simulink model "d"  (R2022b)
settings: Solver=ode4  StartTime=0.0  StopTime=inf  FixedStep=0.002  RelTol=1e-3
InitFcn:
  | init; % init script
values from neighbouring files (symbols this model uses):
  attitude_m0 = [theta_m0; psi_m0]    [init.m]
  attitude_t0 = [theta_t0; psi_t0]    [init.m]
  d_state_m = T_VG_m'*[V_m0;0;0;]    [init.m]
  d_state_t = T_VG_t'*[V_t0;0;0;]    [init.m]
  K_epsilon = k_LOS(1)    [init.m]
  K_sigma = k_LOS(1)    [init.m]
  state_m0 = [x_m0; y_m0; z_m0]    [init.m]
  state_t0 = [x_t0; y_t0; z_t0]    [init.m]
libraries: simulink x1
settings Model: Creator=Ali  LastModifiedBy=Ali

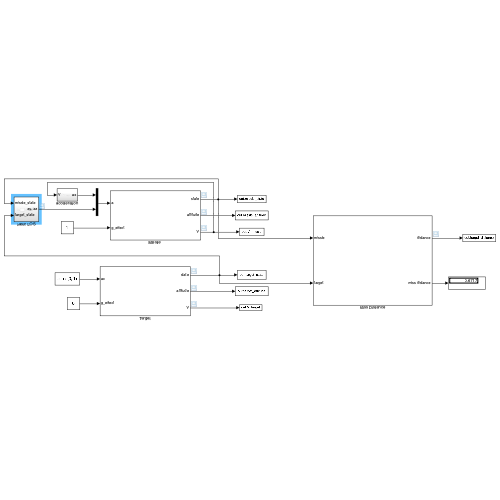
[thumbnail: Simulink's stored preview of the top-level diagram]
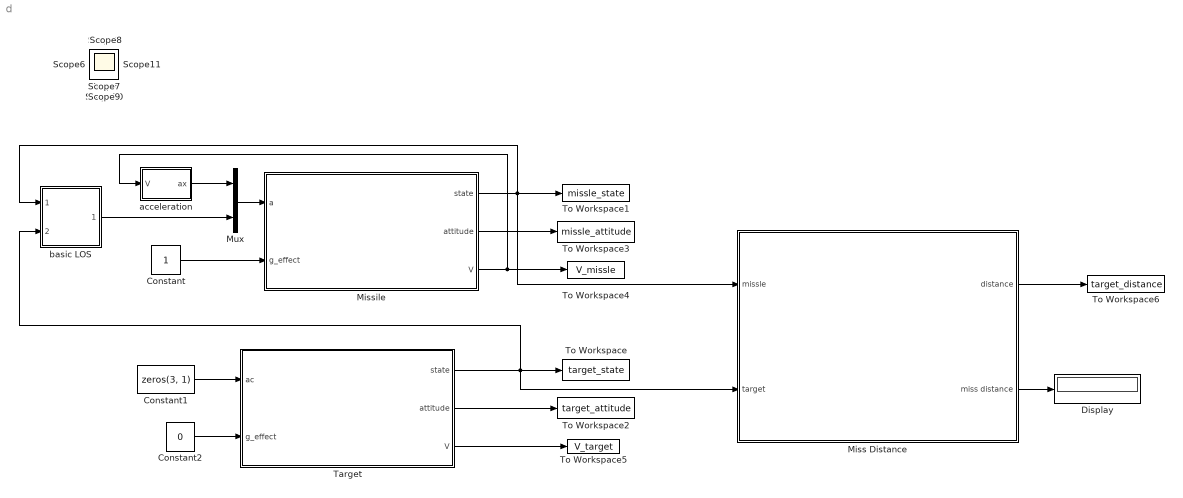
== system d ==
  Constant : Constant
  Constant1 : Constant  Value=zeros(3, 1)
  Constant2 : Constant  Value=0
  Display : Display
  Miss Distance : Subsystem
  "Missile " : Subsystem
  Mux : Mux  Inputs=2
  Target : Subsystem
  To Workspace : ToWorkspace  VariableName=target_state  SaveFormat=Timeseries  SampleTime=-1
      settings: Save2DSignal=2-D array (concatenate along first dimension)
  To Workspace1 : ToWorkspace  VariableName=missle_state  SaveFormat=Timeseries  SampleTime=-1
      settings: Save2DSignal=2-D array (concatenate along first dimension)
  To Workspace2 : ToWorkspace  VariableName=target_attitude  SaveFormat=Timeseries  SampleTime=-1
      settings: Save2DSignal=2-D array (concatenate along first dimension)
  To Workspace3 : ToWorkspace  VariableName=missle_attitude  SaveFormat=Timeseries  SampleTime=-1
      settings: Save2DSignal=2-D array (concatenate along first dimension)
  To Workspace4 : ToWorkspace  VariableName=V_missle  SaveFormat=Timeseries  SampleTime=-1
      settings: Save2DSignal=2-D array (concatenate along first dimension)
  To Workspace5 : ToWorkspace  VariableName=V_target  SaveFormat=Timeseries  SampleTime=-1
      settings: Save2DSignal=2-D array (concatenate along first dimension)
  To Workspace6 : ToWorkspace  VariableName=target_distance  SaveFormat=Timeseries  SampleTime=-1
      settings: Save2DSignal=2-D array (concatenate along first dimension)
  acceleration : Subsystem
  basic LOS : Subsystem
  Scope{,1,6..11} (8 alike) : Scope
  wires:
  Constant/1 -> "Missile "/2(g_effect)
  "Missile "/3(V) -> acceleration/1(V), To Workspace4/1
  Constant1/1 -> Target/1(ac)
  Constant2/1 -> Target/2(g_effect)
  "Missile "/1(state) -> basic LOS/1(missle_state), Miss Distance/1(missle), To Workspace1/1
  "Missile "/2(attitude) -> To Workspace3/1
  Target/1(state) -> basic LOS/2(target_state), Miss Distance/2(target), To Workspace/1
  Target/2(attitude) -> To Workspace2/1
  Target/3(V) -> To Workspace5/1
  Miss Distance/1(distance) -> To Workspace6/1
  Miss Distance/2(miss distance) -> Display/1
  acceleration/1(ax) -> Mux/1
  basic LOS/1("ay, az") -> Mux/2
  Mux/1 -> "Missile "/1(a)

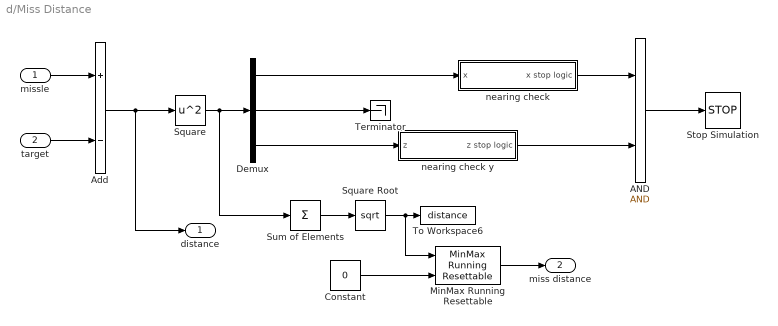
== system d/Miss Distance ==
  missle : Inport
  target : Inport  Port=2
  AND : Logic  IconShape=distinctive  AllPortsSameDT=off  OutDataTypeStr=boolean
  Add : Sum  Inputs=+-
  Constant : Constant  Value=0
  Demux : Demux  Outputs=3
  MinMax Running Resettable : simulink/Math Operations/MinMax Running Resettable  Function=min  vinit=inf
  Square : Math  Operator=square
  Square Root : Sqrt
  Stop Simulation : Stop
  Sum of Elements : Sum  Inputs=+
  Terminator : Terminator
  To Workspace6 : ToWorkspace  VariableName=distance  SaveFormat=Timeseries  SampleTime=-1
      settings: Save2DSignal=2-D array (concatenate along first dimension)
  nearing check : Subsystem
  nearing check y : Subsystem
  distance : Outport
  miss distance : Outport  Port=2
  wires:
  missle/1 -> Add/1
  Add/1 -> distance/1, Square/1
  target/1 -> Add/2
  Square/1 -> Sum of Elements/1, Demux/1
  nearing check/1(x stop logic) -> AND/1
  AND/1 -> Stop Simulation/1
  Demux/2 -> Terminator/1
  nearing check y/1(z stop logic) -> AND/2
  Sum of Elements/1 -> Square Root/1
  Square Root/1 -> MinMax Running Resettable/1, To Workspace6/1
  Demux/3 -> nearing check y/1(z)
  Demux/1 -> nearing check/1(x)
  Constant/1 -> MinMax Running Resettable/2
  MinMax Running Resettable/1 -> miss distance/1

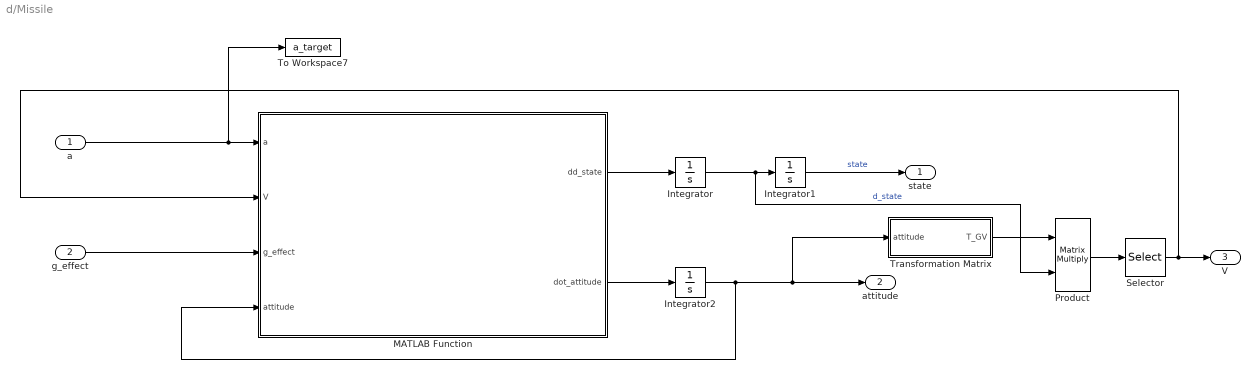
== system d/Missile  ==
  a : Inport
  g_effect : Inport  Port=2
  Integrator : Integrator  InitialCondition=d_state_m
  Integrator1 : Integrator  InitialCondition=state_m0
  Integrator2 : Integrator  InitialCondition=attitude_m0
  MATLAB Function : MATLAB Function  TreatAsAtomicUnit=on
  Product : Product  Multiplication=Matrix(*)
  Selector : Selector  InputPortWidth=3  IndexOptions=Index vector (dialog)  Indices=[1]  OutputSizes=1
  To Workspace7 : ToWorkspace  VariableName=a_target  SampleTime=-1
  Transformation Matrix : MATLAB Function  TreatAsAtomicUnit=on
  state : Outport
  attitude : Outport  Port=2
  V : Outport  Port=3
  wires:
  MATLAB Function/2(dot_attitude) -> Integrator2/1
  Integrator1/1 -> state/1  "state"
  MATLAB Function/1(dd_state) -> Integrator/1
  g_effect/1 -> MATLAB Function/3(g_effect)
  Integrator/1 -> Product/2, Integrator1/1  "d_state"
  Product/1 -> Selector/1
  Selector/1 -> MATLAB Function/2(V), V/1
  Transformation Matrix/1(T_GV) -> Product/1
  Integrator2/1 -> Transformation Matrix/1(attitude), attitude/1, MATLAB Function/4(attitude)
  a/1 -> To Workspace7/1, MATLAB Function/1(a)

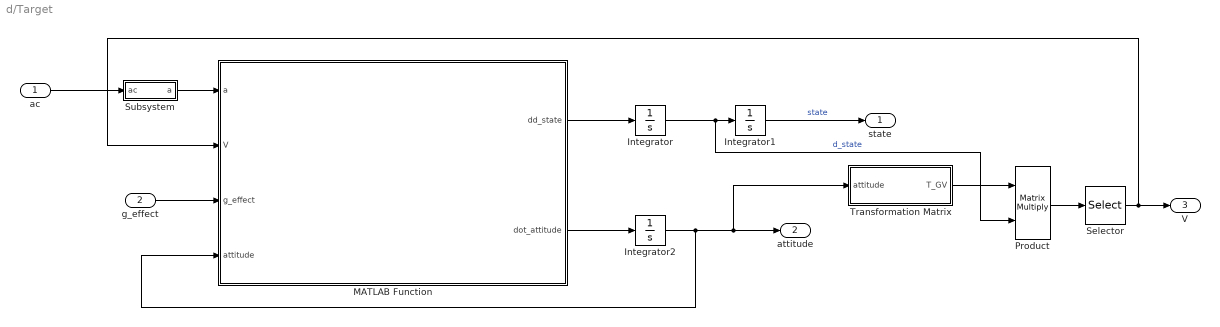
== system d/Target ==
  ac : Inport
  g_effect : Inport  Port=2
  Integrator : Integrator  InitialCondition=d_state_t
  Integrator1 : Integrator  InitialCondition=state_t0
  Integrator2 : Integrator  InitialCondition=attitude_t0
  MATLAB Function : MATLAB Function  TreatAsAtomicUnit=on
  Product : Product  Multiplication=Matrix(*)
  Selector : Selector  InputPortWidth=3  IndexOptions=Index vector (dialog)  Indices=[1]  OutputSizes=1
  Subsystem : Subsystem
  Transformation Matrix : MATLAB Function  TreatAsAtomicUnit=on
  state : Outport
  attitude : Outport  Port=2
  V : Outport  Port=3
  wires:
  MATLAB Function/2(dot_attitude) -> Integrator2/1
  Integrator1/1 -> state/1  "state"
  MATLAB Function/1(dd_state) -> Integrator/1
  g_effect/1 -> MATLAB Function/3(g_effect)
  Integrator/1 -> Product/2, Integrator1/1  "d_state"
  Integrator2/1 -> MATLAB Function/4(attitude), Transformation Matrix/1(attitude), attitude/1
  Product/1 -> Selector/1
  Selector/1 -> MATLAB Function/2(V), V/1
  Transformation Matrix/1(T_GV) -> Product/1
  ac/1 -> Subsystem/1(ac)
  Subsystem/1(a) -> MATLAB Function/1(a)

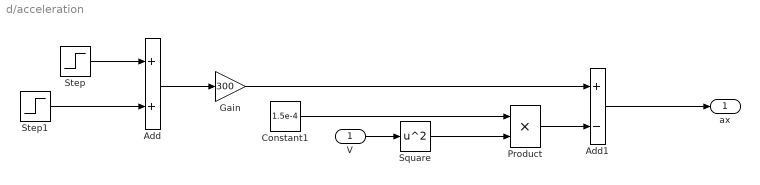
== system d/acceleration ==
  V : Inport
  Add : Sum
  Add1 : Sum  Inputs=+-
  Constant1 : Constant  Value=1.5e-4
  Gain : Gain  Gain=300
  Product : Product
  Square : Math  Operator=square
  Step : Step  Time=3  After=-1  SampleTime=0
  Step1 : Step  Time=0  SampleTime=0
  ax : Outport
  wires:
  V/1 -> Square/1
  Step/1 -> Add/1
  Square/1 -> Product/2
  Constant1/1 -> Product/1
  Add1/1 -> ax/1
  Step1/1 -> Add/2
  Gain/1 -> Add1/1
  Add/1 -> Gain/1
  Product/1 -> Add1/2

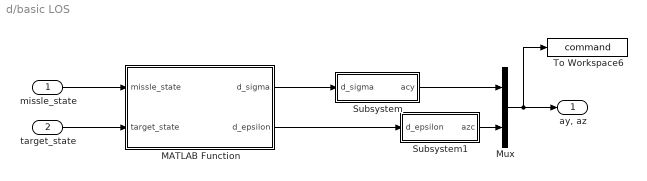
== system d/basic LOS ==
  missle_state : Inport
  target_state : Inport  Port=2
  MATLAB Function : MATLAB Function  TreatAsAtomicUnit=on
  Mux : Mux  Inputs=2
  Subsystem : Subsystem
  Subsystem1 : Subsystem
  To Workspace6 : ToWorkspace  VariableName=command  SaveFormat=Timeseries  SampleTime=-1
      settings: Save2DSignal=2-D array (concatenate along first dimension)
  "ay, az" : Outport
  wires:
  missle_state/1 -> MATLAB Function/1(missle_state)
  Mux/1 -> To Workspace6/1, "ay, az"/1
  target_state/1 -> MATLAB Function/2(target_state)
  MATLAB Function/1(d_sigma) -> Subsystem/1(d_sigma)
  Subsystem/1(acy) -> Mux/1
  MATLAB Function/2(d_epsilon) -> Subsystem1/1(d_epsilon)
  Subsystem1/1(azc) -> Mux/2

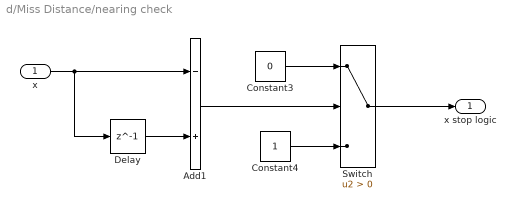
== system d/Miss Distance/nearing check ==
  x : Inport
  Add1 : Sum  Inputs=-+
  Constant3 : Constant  Value=0
  Constant4 : Constant
  Delay : Delay  DelayLength=1  InitialCondition=inf
  Switch : Switch  Criteria=u2 > Threshold  SaturateOnIntegerOverflow=off  InputSameDT=off
  x stop logic : Outport
  wires:
  Switch/1 -> x stop logic/1
  Constant3/1 -> Switch/1
  Constant4/1 -> Switch/3
  x/1 -> Delay/1, Add1/1
  Add1/1 -> Switch/2
  Delay/1 -> Add1/2

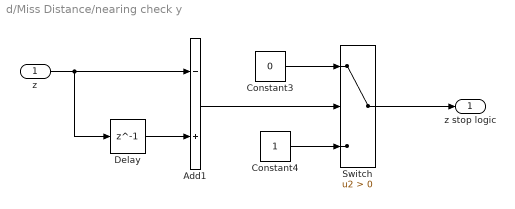
== system d/Miss Distance/nearing check y ==
  z : Inport
  Add1 : Sum  Inputs=-+
  Constant3 : Constant  Value=0
  Constant4 : Constant
  Delay : Delay  DelayLength=1  InitialCondition=inf
  Switch : Switch  Criteria=u2 > Threshold  SaturateOnIntegerOverflow=off  InputSameDT=off
  z stop logic : Outport
  wires:
  Delay/1 -> Add1/2
  Add1/1 -> Switch/2
  z/1 -> Add1/1, Delay/1
  Constant4/1 -> Switch/3
  Constant3/1 -> Switch/1
  Switch/1 -> z stop logic/1

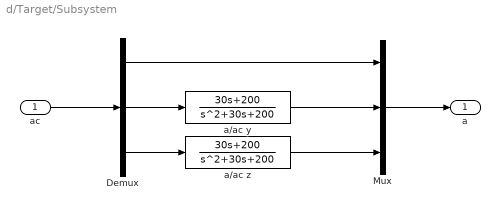
== system d/Target/Subsystem ==
  ac : Inport
  Demux : Demux  Outputs=3
  Mux : Mux  Inputs=3
  a/ac y : TransferFcn  Numerator=[30 200]  Denominator=[1 30 200]
  a/ac z : TransferFcn  Numerator=[30 200]  Denominator=[1 30 200]
  a : Outport
  wires:
  ac/1 -> Demux/1
  Demux/3 -> a/ac z/1
  Demux/2 -> a/ac y/1
  Demux/1 -> Mux/1
  a/ac y/1 -> Mux/2
  a/ac z/1 -> Mux/3
  Mux/1 -> a/1

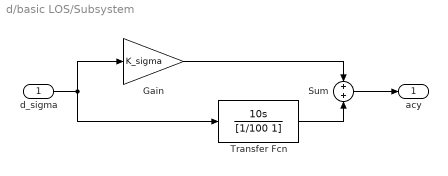
== system d/basic LOS/Subsystem ==
  d_sigma : Inport
  Gain : Gain  Gain=K_sigma
  Sum : Sum  Inputs=+|+
  Transfer Fcn : TransferFcn  Numerator=[10 0]  Denominator=[1/100 1]
  acy : Outport
  wires:
  d_sigma/1 -> Gain/1, Transfer Fcn/1
  Transfer Fcn/1 -> Sum/2
  Sum/1 -> acy/1
  Gain/1 -> Sum/1

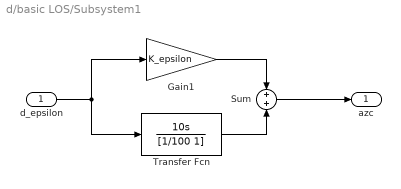
== system d/basic LOS/Subsystem1 ==
  d_epsilon : Inport
  Gain1 : Gain  Gain=K_epsilon
  Sum : Sum  Inputs=+|+
  Transfer Fcn : TransferFcn  Numerator=[10 0]  Denominator=[1/100 1]
  azc : Outport
  wires:
  d_epsilon/1 -> Gain1/1, Transfer Fcn/1
  Gain1/1 -> Sum/1
  Transfer Fcn/1 -> Sum/2
  Sum/1 -> azc/1

== matlab function d/Missile /Transformation Matrix ==
  data: attitude input; T_GV output
function T_GV = fcn(attitude)
theta = attitude(1);
psi = attitude(2);

T_GV = [cos(theta)*cos(psi)   cos(theta)*sin(psi)   sin(theta)
            -sin(psi)               cos(psi)            0
        -sin(theta)*cos(psi)  -sin(theta)*sin(psi)   cos(theta) ];

== matlab function d/Missile /MATLAB Function ==
  data: a input; dd_state output; V input; g_effect input; attitude input; dot_attitude output
function [dd_state, dot_attitude] =...
    fcn(a, V, g_effect, attitude)
a_x = a(1);
a_y = a(2);
a_z = a(3);

theta = attitude(1);
psi = attitude(2);
g = 9.81;
g = g*g_effect;

ddot_x = a_x*cos(theta)*cos(psi) - a_y*sin(psi) - a_z*sin(theta)*cos(psi);
ddot_y = a_x*cos(theta)*sin(psi) + a_y*cos(psi) - a_z*sin(theta)*sin(psi);
ddot_z = a_x*sin(theta) + a_z*cos(theta) - g;

dd_state = [ddot_x; ddot_y; ddot_z];

dot_theta = (a_z - g*cos(theta)) / V;
dot_psi   = a_y / (V*cos(theta));

dot_attitude = [dot_theta; dot_psi];

== matlab function d/Target/MATLAB Function ==
  data: a input; dd_state output; V input; g_effect input; attitude input; dot_attitude output
function [dd_state, dot_attitude] =...
    fcn(a, V, g_effect, attitude)
a_x = a(1);
a_y = a(2);
a_z = a(3);

theta = attitude(1);
psi = attitude(2);
g = 9.81;
g = g*g_effect;

ddot_x = a_x*cos(theta)*cos(psi) - a_y*sin(psi) - a_z*sin(theta)*cos(psi);
ddot_y = a_x*cos(theta)*sin(psi) + a_y*cos(psi) - a_z*sin(theta)*sin(psi);
ddot_z = a_x*sin(theta) + a_z*cos(theta) - g;

dd_state = [ddot_x; ddot_y; ddot_z];

dot_theta = (a_z - g*cos(theta)) / V;
dot_psi   = a_y / (V*cos(theta));

dot_attitude = [dot_theta; dot_psi];

== matlab function d/Target/Transformation Matrix ==
  data: attitude input; T_GV output
function T_GV = fcn(attitude)
theta = attitude(1);
psi = attitude(2);

T_VG = [cos(theta)*cos(psi)   cos(theta)*sin(psi)   sin(theta)
            -sin(psi)               cos(psi)            0
        -sin(theta)*cos(psi)  -sin(theta)*sin(psi)   cos(theta) ];

T_GV = T_VG';

== matlab function d/basic LOS/MATLAB Function ==
  data: d_sigma output; missle_state input; d_epsilon output; target_state input
function [d_sigma, d_epsilon] = fcn(missle_state, target_state)

[sigma_m, epsilon_m] = angle_calculator(missle_state);
[sigma_t, epsilon_t] = angle_calculator(target_state);

d_epsilon = norm(missle_state)*(epsilon_t - epsilon_m);
d_sigma = norm(missle_state)*(sigma_t - sigma_m)*cos(epsilon_t);

end


function [sigma, epsilon] = angle_calculator(state)
    if norm(state) == 0
        epsilon = 0;
        sigma = 0;
        return
    end
    epsilon = asin(state(3)/norm(state));
    sigma = atan2(state(2),state(1));
end
